simulink library "mag_block_visual"  (R2025b)
settings: Solver=VariableStepAuto  StartTime=0.0  StopTime=10.0  RelTol=1e-3
values from neighbouring files (symbols this model uses):
  Mag = evalin('base', 'Mag')    [test_mag_block_visual_compile.m]    (also in test_mag_model.m)
  Sim = evalin('base', 'Sim')    [casper_mag_step.m]    (also in test_mag_model.m)
settings Model: Creator=Ashwin  LastModifiedBy=Ashwin

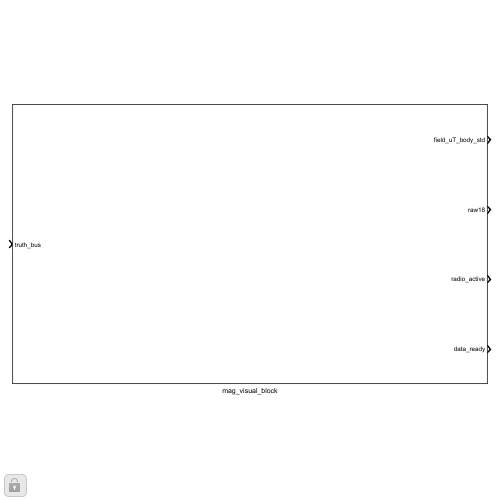
[thumbnail: Simulink's stored preview of the top-level diagram]
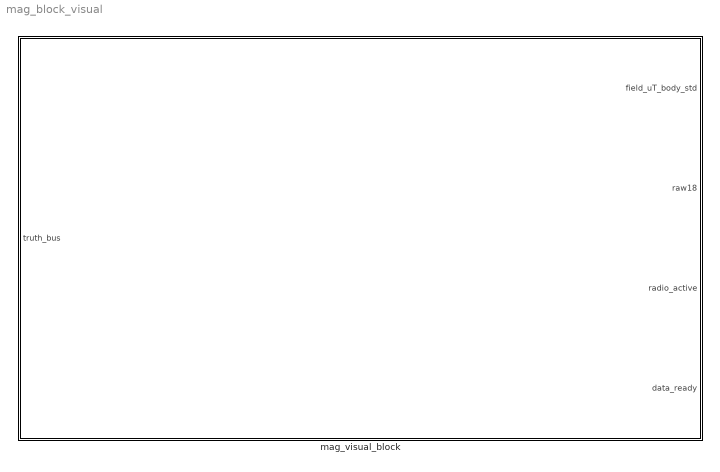
== system mag_block_visual ==
  mag_visual_block : Subsystem

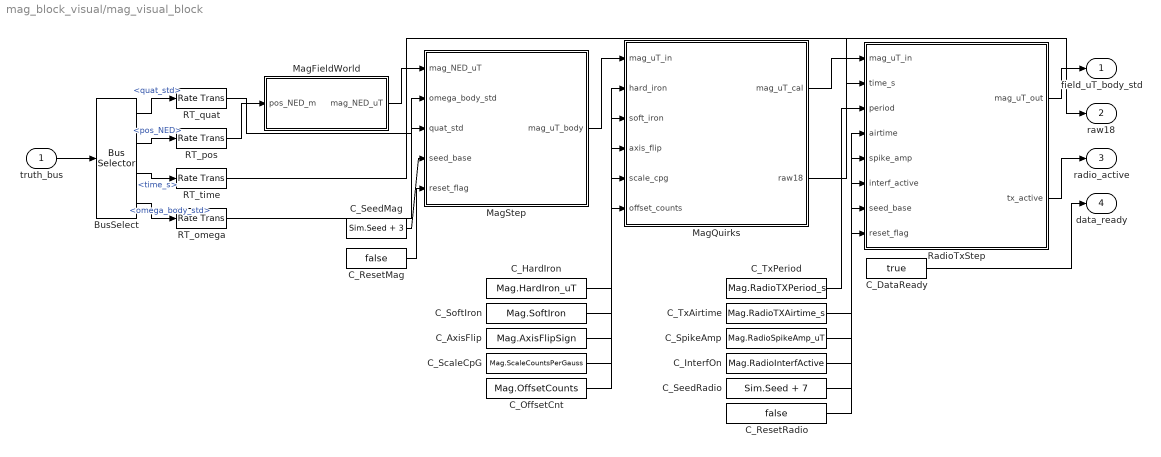
== system mag_block_visual/mag_visual_block ==
  truth_bus : Inport  OutDataTypeStr=Bus: SensorInputBus
  BusSelect : BusSelector  OutputSignals=quat_std,pos_NED,time_s,omega_body_std
  C_AxisFlip : Constant  Value=Mag.AxisFlipSign  SampleTime=1/Mag.Rate_Hz
  C_DataReady : Constant  Value=true  OutDataTypeStr=boolean  SampleTime=1/Mag.Rate_Hz
  C_HardIron : Constant  Value=Mag.HardIron_uT  SampleTime=1/Mag.Rate_Hz
  C_InterfOn : Constant  Value=Mag.RadioInterfActive  OutDataTypeStr=boolean  SampleTime=1/Mag.Rate_Hz
  C_OffsetCnt : Constant  Value=Mag.OffsetCounts  SampleTime=1/Mag.Rate_Hz
  C_ResetMag : Constant  Value=false  OutDataTypeStr=boolean  SampleTime=1/Mag.Rate_Hz
  C_ResetRadio : Constant  Value=false  OutDataTypeStr=boolean  SampleTime=1/Mag.Rate_Hz
  C_ScaleCpG : Constant  Value=Mag.ScaleCountsPerGauss  SampleTime=1/Mag.Rate_Hz
  C_SeedMag : Constant  Value=Sim.Seed + 3  SampleTime=1/Mag.Rate_Hz
  C_SeedRadio : Constant  Value=Sim.Seed + 7  SampleTime=1/Mag.Rate_Hz
  C_SoftIron : Constant  Value=Mag.SoftIron  SampleTime=1/Mag.Rate_Hz
  C_SpikeAmp : Constant  Value=Mag.RadioSpikeAmp_uT  SampleTime=1/Mag.Rate_Hz
  C_TxAirtime : Constant  Value=Mag.RadioTXAirtime_s  SampleTime=1/Mag.Rate_Hz
  C_TxPeriod : Constant  Value=Mag.RadioTXPeriod_s  SampleTime=1/Mag.Rate_Hz
  MagFieldWorld : MATLAB Function  TreatAsAtomicUnit=on
  MagQuirks : MATLAB Function  TreatAsAtomicUnit=on
  MagStep : MATLAB Function  TreatAsAtomicUnit=on
  RT_omega : RateTransition  OutPortSampleTime=1/Mag.Rate_Hz
  RT_pos : RateTransition  OutPortSampleTime=1/Mag.Rate_Hz
  RT_quat : RateTransition  OutPortSampleTime=1/Mag.Rate_Hz
  RT_time : RateTransition  OutPortSampleTime=1/Mag.Rate_Hz
  RadioTxStep : MATLAB Function  TreatAsAtomicUnit=on
  field_uT_body_std : Outport
  raw18 : Outport  Port=2
  radio_active : Outport  Port=3
  data_ready : Outport  Port=4
  wires:
  truth_bus/1 -> BusSelect/1
  BusSelect/1 -> RT_quat/1  "<quat_std>"
  BusSelect/2 -> RT_pos/1  "<pos_NED>"
  BusSelect/3 -> RT_time/1  "<time_s>"
  BusSelect/4 -> RT_omega/1  "<omega_body_std>"
  RT_pos/1 -> MagFieldWorld/1(pos_NED_m)
  MagFieldWorld/1(mag_NED_uT) -> MagStep/1(mag_NED_uT)
  RT_omega/1 -> MagStep/2(omega_body_std)
  RT_quat/1 -> MagStep/3(quat_std)
  C_SeedMag/1 -> MagStep/4(seed_base)
  C_ResetMag/1 -> MagStep/5(reset_flag)
  MagStep/1(mag_uT_body) -> MagQuirks/1(mag_uT_in)
  C_HardIron/1 -> MagQuirks/2(hard_iron)
  C_SoftIron/1 -> MagQuirks/3(soft_iron)
  C_AxisFlip/1 -> MagQuirks/4(axis_flip)
  C_ScaleCpG/1 -> MagQuirks/5(scale_cpg)
  C_OffsetCnt/1 -> MagQuirks/6(offset_counts)
  MagQuirks/1(mag_uT_cal) -> RadioTxStep/1(mag_uT_in)
  RT_time/1 -> RadioTxStep/2(time_s)
  C_TxPeriod/1 -> RadioTxStep/3(period)
  C_TxAirtime/1 -> RadioTxStep/4(airtime)
  C_SpikeAmp/1 -> RadioTxStep/5(spike_amp)
  C_InterfOn/1 -> RadioTxStep/6(interf_active)
  C_SeedRadio/1 -> RadioTxStep/7(seed_base)
  C_ResetRadio/1 -> RadioTxStep/8(reset_flag)
  RadioTxStep/1(mag_uT_out) -> field_uT_body_std/1
  MagQuirks/2(raw18) -> raw18/1
  RadioTxStep/2(tx_active) -> radio_active/1
  C_DataReady/1 -> data_ready/1

== matlab function mag_block_visual/mag_visual_block/MagStep ==
  data: mag_NED_uT input; mag_uT_body output; omega_body_std input; quat_std input; seed_base input; reset_flag input
function mag_uT_body = fcn(mag_NED_uT, omega_body_std, quat_std, seed_base, reset_flag)
coder.extrinsic('casper_mag_step');
mag_uT_body = zeros(3,1);
tmp_row = zeros(1,3);
[tmp_row, ~] = casper_mag_step(mag_NED_uT(:).', omega_body_std(:).', quat_std(:).', double(seed_base), logical(reset_flag));
mag_uT_body = tmp_row(:);
end

== matlab function mag_block_visual/mag_visual_block/MagFieldWorld ==
  data: pos_NED_m input; mag_NED_uT output
function mag_NED_uT = fcn(pos_NED_m)
%#codegen
mag_NED_uT = casper_mag_field_world(pos_NED_m);
end

== matlab function mag_block_visual/mag_visual_block/MagQuirks ==
  data: mag_uT_in input; mag_uT_cal output; hard_iron input; soft_iron input; axis_flip input; scale_cpg input; offset_counts input; raw18 output
function [mag_uT_cal, raw18] = fcn(mag_uT_in, hard_iron, soft_iron, axis_flip, scale_cpg, offset_counts)
%#codegen
[mag_uT_cal, raw18] = casper_mag_quirks(mag_uT_in(:), hard_iron(:), soft_iron, axis_flip(:), scale_cpg, offset_counts);
end

== matlab function mag_block_visual/mag_visual_block/RadioTxStep ==
  data: mag_uT_in input; mag_uT_out output; time_s input; period input; airtime input; spike_amp input; interf_active input; seed_base input; reset_flag input; tx_active output
function [mag_uT_out, tx_active] = fcn(mag_uT_in, time_s, period, airtime, spike_amp, interf_active, seed_base, reset_flag)
coder.extrinsic('casper_radio_tx_step');
mag_uT_out = zeros(3,1);
tx_active  = false;
[mag_uT_out, tx_active, ~, ~] = casper_radio_tx_step(mag_uT_in(:), double(time_s), double(period), double(airtime), double(spike_amp), logical(interf_active), double(seed_base), logical(reset_flag));
end
